simulink model "simulate_OFDM_basebandModulatorDemodulator"  (R2017a)
settings: Solver=VariableStepAuto  StartTime=0.0  StopTime=.01  RelTol=1e-3
InitFcn:
  | Ts = 1/1000; % symbol time in serial data stream
  | N = 4; % number of orthogonal carriers
  | T = N*Ts; % symbol time in parallel data stream
libraries: commfilt2 x8, dspsrcs4 x8, commdigbbndpm3 x2, commrandsrc3 x1, dspindex x1
settings Model: Creator=prust  LastModifiedBy=prust

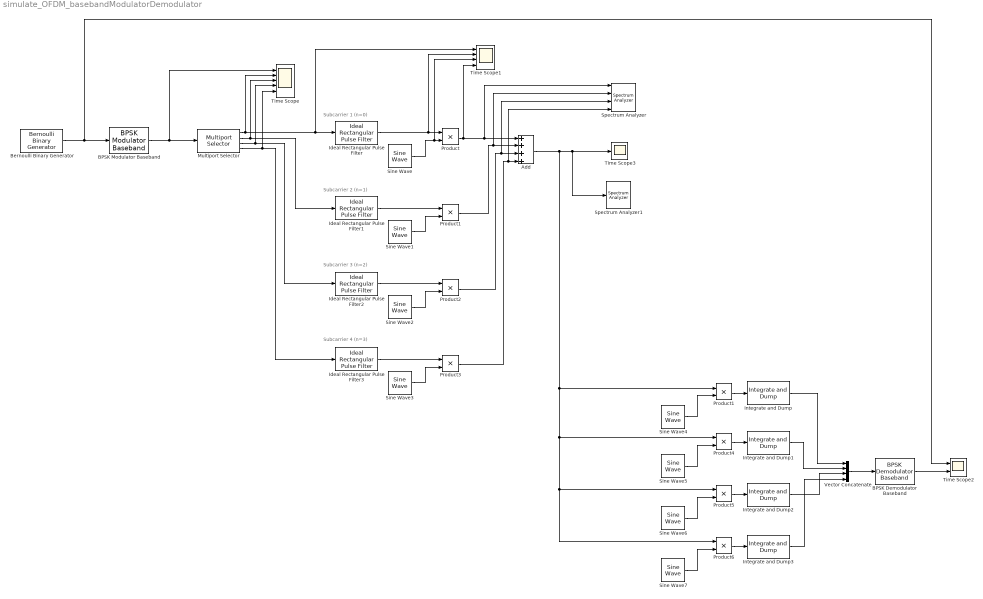
== system simulate_OFDM_basebandModulatorDemodulator ==
  note: Subcarrier 4 (n=3)
  note: Subcarrier 3 (n=2)
  note: Subcarrier 2 (n=1)
  note: Subcarrier 1 (n=0)
  Add : Sum  Inputs=4
  BPSK Demodulator Baseband : commdigbbndpm3/BPSK Demodulator Baseband  DecType=Hard decision  VarSource=Dialog  Variance=1  Ph=0  outDtype=Inherit via internal rule  derotateFactorWordLen=16  derotateFactorDataTypeStr=Inherit: Same word length as input  derotateFactorLastDataTypeStr=Inherit: Same word length as input
  BPSK Modulator Baseband : commdigbbndpm3/BPSK Modulator Baseband  Ph=0  outDtype=double  outWordLen=16  outUDDataType=sfix(16)  outFracLenMode=Best precision  outFracLen=15  outDataTypeStr=double  outLastDataTypeStr=double
  Bernoulli Binary Generator : commrandsrc3/Bernoulli Binary Generator  ProbabilityOfZero=0.5  SeedSource=Auto  Seed=0  SampleTime=Ts  SamplesPerFrame=4  OutputDataType=double  SimulateUsing=Interpreted execution
  Ideal Rectangular Pulse Filter{,1..3} (4 alike) : commfilt2/Ideal Rectangular Pulse Filter  pulseLen=8  pulseDelay=0  InputProcessing=Columns as channels (frame based)  RateOptions=Enforce single-rate processing  sampMode=Mute  normCheck=off  normMode=Sum of samples  filterGain=1  saveAsFlag=0  roundingMode=Floor  overflowMode=off  firstCoeffDataTypeStr=Inherit: Same word length as input  firstCoeffMin=[]  firstCoeffMax=[]  firstCoeffLastDataTypeStr=Inherit: Same word length as input  outputDataTypeStr=Inherit: Same as accumulator  outputMin=[]  outputMax=[]  outputLastDataTypeStr=Inherit: Same as accumulator
      settings: SourceProductName=Communications System Toolbox  SourceProductBaseCode=CM
  Integrate and Dump{,1..3} (4 alike) : commfilt2/Integrate and Dump  obssamples=8  offsetsamples=0  nodump=off  roundingMode=Floor  overflowMode=off  outputDataTypeStr=Inherit: Same as accumulator  outputLastDataTypeStr=Inherit: Same as accumulator
      settings: SourceProductName=Communications System Toolbox
  Multiport Selector : dspindex/Multiport Selector  rowsOrCols=Rows  idxCellArray={ 1, 2, 3, 4 }  idxErrMode=Clip Index
  Product{,1..6} (7 alike) : Product
  "Product1 " : Product
  Sine Wave : dspsrcs4/Sine Wave  Amplitude=1  Frequency=-375  Phase=0  SampleMode=Discrete  OutComplex=Complex  CompMethod=Trigonometric fcn  TableSize=Speed  SampleTime=T/8  SamplesPerFrame=8  ResetState=Restart at time zero  OutputFrames=off  dataType=double  wordLen=16  udDataType=sfix(16)  fracBitsMode=Best precision  numFracBits=15  OutDataTypeStr=double  LastOutDataTypeStr=double
  Sine Wave1 : dspsrcs4/Sine Wave  Amplitude=1  Frequency=-125  Phase=0  SampleMode=Discrete  OutComplex=Complex  CompMethod=Trigonometric fcn  TableSize=Speed  SampleTime=T/8  SamplesPerFrame=8  ResetState=Restart at time zero  OutputFrames=off  dataType=double  wordLen=16  udDataType=sfix(16)  fracBitsMode=Best precision  numFracBits=15  OutDataTypeStr=double  LastOutDataTypeStr=double
  Sine Wave2 : dspsrcs4/Sine Wave  Amplitude=1  Frequency=125  Phase=0  SampleMode=Discrete  OutComplex=Complex  CompMethod=Trigonometric fcn  TableSize=Speed  SampleTime=T/8  SamplesPerFrame=8  ResetState=Restart at time zero  OutputFrames=off  dataType=double  wordLen=16  udDataType=sfix(16)  fracBitsMode=Best precision  numFracBits=15  OutDataTypeStr=double  LastOutDataTypeStr=double
  Sine Wave3 : dspsrcs4/Sine Wave  Amplitude=1  Frequency=375  Phase=0  SampleMode=Discrete  OutComplex=Complex  CompMethod=Trigonometric fcn  TableSize=Speed  SampleTime=T/8  SamplesPerFrame=8  ResetState=Restart at time zero  OutputFrames=off  dataType=double  wordLen=16  udDataType=sfix(16)  fracBitsMode=Best precision  numFracBits=15  OutDataTypeStr=double  LastOutDataTypeStr=double
  Sine Wave4 : dspsrcs4/Sine Wave  Amplitude=1  Frequency=375  Phase=0  SampleMode=Discrete  OutComplex=Complex  CompMethod=Trigonometric fcn  TableSize=Speed  SampleTime=T/8  SamplesPerFrame=8  ResetState=Restart at time zero  OutputFrames=off  dataType=double  wordLen=16  udDataType=sfix(16)  fracBitsMode=Best precision  numFracBits=15  OutDataTypeStr=double  LastOutDataTypeStr=double
  Sine Wave5 : dspsrcs4/Sine Wave  Amplitude=1  Frequency=125  Phase=0  SampleMode=Discrete  OutComplex=Complex  CompMethod=Trigonometric fcn  TableSize=Speed  SampleTime=T/8  SamplesPerFrame=8  ResetState=Restart at time zero  OutputFrames=off  dataType=double  wordLen=16  udDataType=sfix(16)  fracBitsMode=Best precision  numFracBits=15  OutDataTypeStr=double  LastOutDataTypeStr=double
  Sine Wave6 : dspsrcs4/Sine Wave  Amplitude=1  Frequency=-125  Phase=0  SampleMode=Discrete  OutComplex=Complex  CompMethod=Trigonometric fcn  TableSize=Speed  SampleTime=T/8  SamplesPerFrame=8  ResetState=Restart at time zero  OutputFrames=off  dataType=double  wordLen=16  udDataType=sfix(16)  fracBitsMode=Best precision  numFracBits=15  OutDataTypeStr=double  LastOutDataTypeStr=double
  Sine Wave7 : dspsrcs4/Sine Wave  Amplitude=1  Frequency=-375  Phase=0  SampleMode=Discrete  OutComplex=Complex  CompMethod=Trigonometric fcn  TableSize=Speed  SampleTime=T/8  SamplesPerFrame=8  ResetState=Restart at time zero  OutputFrames=off  dataType=double  wordLen=16  udDataType=sfix(16)  fracBitsMode=Best precision  numFracBits=15  OutDataTypeStr=double  LastOutDataTypeStr=double
  Spectrum Analyzer : SpectrumAnalyzer  NumInputPorts=4
  Spectrum Analyzer1 : SpectrumAnalyzer
  Time Scope : Scope  NumInputPorts=5
  Time Scope1 : Scope  NumInputPorts=4
  Time Scope2 : Scope  NumInputPorts=2
  Time Scope3 : Scope
  Vector Concatenate : Concatenate  NumInputs=4
  wires:
  Bernoulli Binary Generator/1 -> Time Scope2/1, BPSK Modulator Baseband/1
  Sine Wave1/1 -> "Product1 "/2
  Multiport Selector/2 -> Time Scope/3, Ideal Rectangular Pulse Filter1/1
  Multiport Selector/1 -> Time Scope/2, Time Scope1/1, Ideal Rectangular Pulse Filter/1
  Sine Wave/1 -> Time Scope1/3, Product/2
  Multiport Selector/3 -> Time Scope/4, Ideal Rectangular Pulse Filter2/1
  Sine Wave2/1 -> Product2/2
  Sine Wave3/1 -> Product3/2
  Multiport Selector/4 -> Time Scope/5, Ideal Rectangular Pulse Filter3/1
  Product/1 -> Time Scope1/4, Add/1, Spectrum Analyzer/1
  "Product1 "/1 -> Spectrum Analyzer/2, Add/2
  Product2/1 -> Spectrum Analyzer/3, Add/3
  Product3/1 -> Spectrum Analyzer/4, Add/4
  Ideal Rectangular Pulse Filter/1 -> Time Scope1/2, Product/1
  Ideal Rectangular Pulse Filter1/1 -> "Product1 "/1
  Ideal Rectangular Pulse Filter2/1 -> Product2/1
  Ideal Rectangular Pulse Filter3/1 -> Product3/1
  BPSK Modulator Baseband/1 -> Time Scope/1, Multiport Selector/1
  Sine Wave4/1 -> Product1/2
  Product1/1 -> Integrate and Dump/1
  Product4/1 -> Integrate and Dump1/1
  Sine Wave5/1 -> Product4/2
  Product5/1 -> Integrate and Dump2/1
  Sine Wave6/1 -> Product5/2
  Product6/1 -> Integrate and Dump3/1
  Sine Wave7/1 -> Product6/2
  Add/1 -> Product6/1, Product5/1, Product4/1, Product1/1, Time Scope3/1, Spectrum Analyzer1/1
  Integrate and Dump/1 -> Vector Concatenate/1
  Integrate and Dump1/1 -> Vector Concatenate/2
  Integrate and Dump2/1 -> Vector Concatenate/3
  Integrate and Dump3/1 -> Vector Concatenate/4
  Vector Concatenate/1 -> BPSK Demodulator Baseband/1
  BPSK Demodulator Baseband/1 -> Time Scope2/2
